simulink model "interactive_sample"  (Simulink 7.6)
settings: Solver=ode3  SolverMode=SingleTasking  StartTime=0.0  StopTime=inf  FixedStep=0.1  RelTol=1e-3
settings Model: Creator=Victor  LastModifiedBy=Student
settings OptimizationCC: BlockReduction=off  BooleanDataType=off  ExpressionDepthLimit=128
settings DebuggingCC: SaveWithParameterizedLinksMsg=none  SignalResolutionControl=TryResolveAllWithWarning  SolverPrmCheckMsg=none  StateNameClashWarn=none  StrictBusMsg=Warning
settings HardwareCC: TargetUnknown=on
settings CodeAppCC: CustomSymbolStrType=$N$R$M_T
settings GRTTargetCC: TargetFunctionLibrary=NOT IN USE  CombineOutputUpdateFcns=on  CPPClassGenCompliant=on

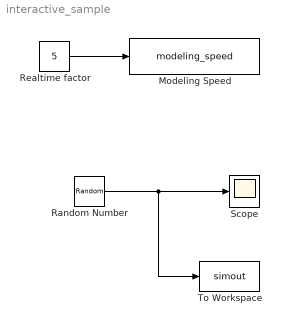
== system interactive_sample ==
  Modeling Speed : S-Function  FunctionName=modeling_speed  EnableBusSupport=off
  Random Number : RandomNumber  Variance=10  SampleTime=0.1
  Realtime factor : Constant  Value=5
  Scope : Scope
      settings: DataFormat=Array
  To Workspace : ToWorkspace  VariableName=simout  SampleTime=-1  SaveFormat=Array
  wires:
  Random Number/1 -> To Workspace/1, Scope/1
  Realtime factor/1 -> Modeling Speed/1
